simulink model "platoon"  (R2023a)
settings: Solver=VariableStepAuto  StartTime=0.0  StopTime=50  RelTol=1e-3
values from neighbouring files (symbols this model uses):
  d_default = 0.5    [prerun.m]
  t_hw = 0.1    [prerun.m]
  td_comm = 0.1    [prerun.m]
  td_comm_leader = ones(n,1)    [prerun.m]
  td_input = 0    [prerun.m]
undefined symbols (not defined in the file or in its folder): sigbuilder_block
libraries: cstblocks x21, slpidlib x2
settings Model: Creator=ritvi  LastModifiedBy=ritvi

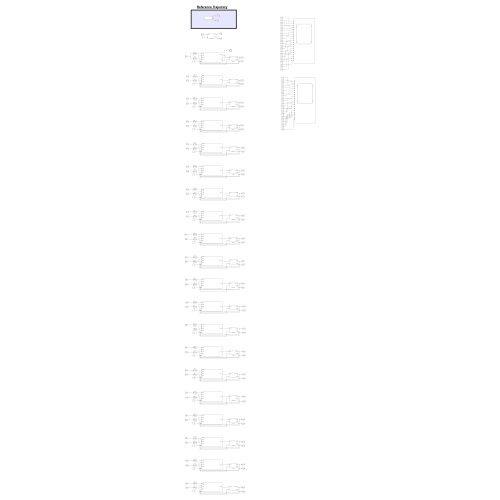
[thumbnail: Simulink's stored preview of the top-level diagram]
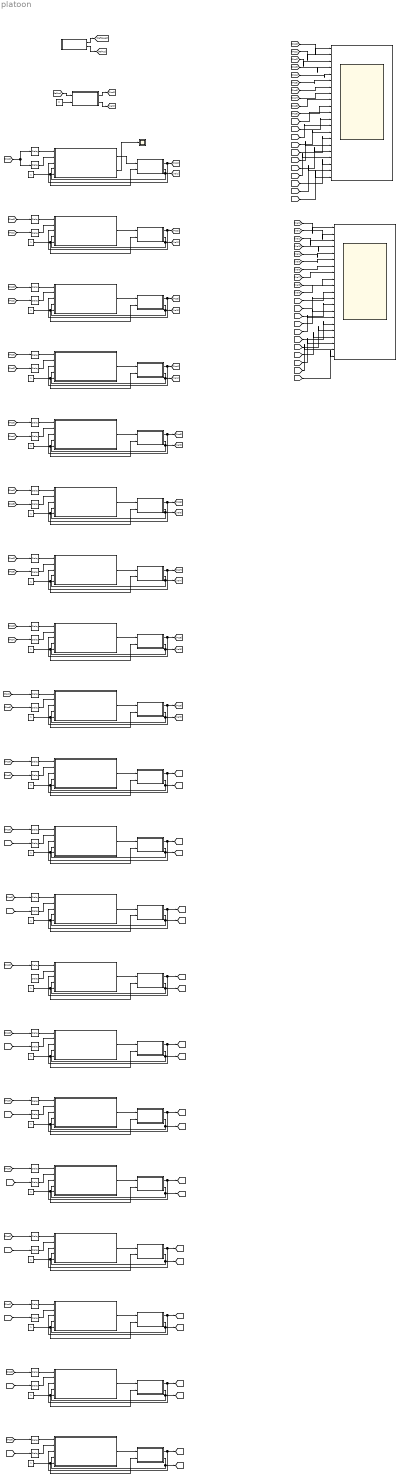
== system platoon ==
  note: Reference Trajectory
  Constant : Constant  Value=0
  Constant{1..20} (20 alike) : Constant
  Scope : Scope  NumInputPorts=21
  Scope1 : Scope  NumInputPorts=21
  Scope2 : Scope
  Subsystem : Subsystem
  Subsystem1 : Subsystem
  Subsystem10 : Subsystem
  Subsystem11 : Subsystem
  Subsystem12 : Subsystem
  Subsystem13 : Subsystem
  Subsystem14 : Subsystem
  Subsystem15 : Subsystem
  Subsystem16 : Subsystem
  Subsystem17 : Subsystem
  Subsystem18 : Subsystem
  Subsystem19 : Subsystem
  Subsystem2 : Subsystem
  Subsystem20 : Subsystem
  Subsystem3 : Subsystem
  Subsystem4 : Subsystem
  Subsystem5 : Subsystem
  Subsystem6 : Subsystem
  Subsystem7 : Subsystem
  Subsystem8 : Subsystem
  Subsystem9 : Subsystem
  Transport Delay{,2,4,6,8,10,12,14,16,18,20,22,24,26,28,30,32,34,36,38} (20 alike) : TransportDelay  DelayTime=td_comm
  Transport Delay1 : TransportDelay  DelayTime=td_comm_leader(1)
  Transport Delay11 : TransportDelay  DelayTime=td_comm_leader(6)
  Transport Delay13 : TransportDelay  DelayTime=td_comm_leader(7)
  Transport Delay15 : TransportDelay  DelayTime=td_comm_leader(8)
  Transport Delay17 : TransportDelay  DelayTime=td_comm_leader(9)
  Transport Delay19 : TransportDelay  DelayTime=td_comm_leader(10)
  Transport Delay21 : TransportDelay  DelayTime=td_comm_leader(11)
  Transport Delay23 : TransportDelay  DelayTime=td_comm_leader(12)
  Transport Delay25 : TransportDelay  DelayTime=td_comm_leader(13)
  Transport Delay27 : TransportDelay  DelayTime=td_comm_leader(14)
  Transport Delay29 : TransportDelay  DelayTime=td_comm_leader(15)
  Transport Delay3 : TransportDelay  DelayTime=td_comm_leader(2)
  Transport Delay31 : TransportDelay  DelayTime=td_comm_leader(16)
  Transport Delay33 : TransportDelay  DelayTime=td_comm_leader(17)
  Transport Delay35 : TransportDelay  DelayTime=td_comm_leader(18)
  Transport Delay37 : TransportDelay  DelayTime=td_comm_leader(19)
  Transport Delay39 : TransportDelay  DelayTime=td_comm_leader(20)
  Transport Delay5 : TransportDelay  DelayTime=td_comm_leader(3)
  Transport Delay7 : TransportDelay  DelayTime=td_comm_leader(4)
  Transport Delay9 : TransportDelay  DelayTime=td_comm_leader(5)
  Vehicle 0 : Subsystem
  Vehicle 1 : Subsystem
  Vehicle 10 : Subsystem
  Vehicle 11 : Subsystem
  Vehicle 12 : Subsystem
  Vehicle 13 : Subsystem
  Vehicle 14 : Subsystem
  Vehicle 15 : Subsystem
  Vehicle 16 : Subsystem
  Vehicle 17 : Subsystem
  Vehicle 18 : Subsystem
  Vehicle 19 : Subsystem
  Vehicle 2 : Subsystem
  Vehicle 20 : Subsystem
  Vehicle 3 : Subsystem
  Vehicle 4 : Subsystem
  Vehicle 5 : Subsystem
  Vehicle 6 : Subsystem
  Vehicle 7 : Subsystem
  Vehicle 8 : Subsystem
  Vehicle 9 : Subsystem
  wires:
  Subsystem1/1(vl) -> [RefSpeed]
  Subsystem1/2(al) -> [RefAcc]
  Subsystem/1(CmdAcc) -> Vehicle 1/1(RefAcc)
  Vehicle 1/1(position) -> [Pos1], Subsystem/3(PosEgo)
  Vehicle 1/2(speed) -> Subsystem/4(VelEgo), [Vel1]
  Constant1/1 -> Vehicle 1/2(i), Subsystem/5(i)
  Transport Delay/1 -> Subsystem/2(PosPred)
  Constant/1 -> Vehicle 0/2(i)
  [RefAcc] -> Vehicle 0/1(RefAcc)
  Vehicle 0/1(position) -> [Pos0]
  Vehicle 0/2(speed) -> [Vel0]
  Transport Delay1/1 -> Subsystem/1(PosLead)
  [Pos0] -> Transport Delay1/1, Transport Delay/1
  [Pos0] -> Transport Delay3/1
  Transport Delay2/1 -> Subsystem2/2(PosPred)
  Subsystem2/1(CmdAcc) -> Vehicle 2/1(RefAcc)
  Vehicle 2/1(position) -> [Pos2], Subsystem2/3(PosEgo)
  Vehicle 2/2(speed) -> Subsystem2/4(VelEgo), [Vel2]
  Constant2/1 -> Vehicle 2/2(i), Subsystem2/5(i)
  Transport Delay3/1 -> Subsystem2/1(PosLead)
  [Pos0] -> Transport Delay5/1
  Transport Delay4/1 -> Subsystem3/2(PosPred)
  Subsystem3/1(CmdAcc) -> Vehicle 3/1(RefAcc)
  Vehicle 3/1(position) -> [Pos3], Subsystem3/3(PosEgo)
  Vehicle 3/2(speed) -> [Vel3], Subsystem3/4(VelEgo)
  Constant3/1 -> Vehicle 3/2(i), Subsystem3/5(i)
  Transport Delay5/1 -> Subsystem3/1(PosLead)
  Vehicle 5/2(speed) -> [Vel5], Subsystem5/4(VelEgo)
  Transport Delay9/1 -> Subsystem5/1(PosLead)
  Subsystem5/1(CmdAcc) -> Vehicle 5/1(RefAcc)
  Vehicle 5/1(position) -> [Pos5], Subsystem5/3(PosEgo)
  Transport Delay8/1 -> Subsystem5/2(PosPred)
  [Pos0] -> Transport Delay9/1
  Transport Delay7/1 -> Subsystem4/1(PosLead)
  [Pos0] -> Transport Delay7/1
  Vehicle 4/2(speed) -> [Vel4], Subsystem4/4(VelEgo)
  Constant5/1 -> Vehicle 5/2(i), Subsystem5/5(i)
  Transport Delay6/1 -> Subsystem4/2(PosPred)
  Constant4/1 -> Vehicle 4/2(i), Subsystem4/5(i)
  Subsystem4/1(CmdAcc) -> Vehicle 4/1(RefAcc)
  Vehicle 4/1(position) -> Subsystem4/3(PosEgo), [Pos4]
  Vehicle 7/2(speed) -> Subsystem7/4(VelEgo), [Vel7]
  Transport Delay13/1 -> Subsystem7/1(PosLead)
  Subsystem7/1(CmdAcc) -> Vehicle 7/1(RefAcc)
  Vehicle 7/1(position) -> [Pos7], Subsystem7/3(PosEgo)
  Transport Delay12/1 -> Subsystem7/2(PosPred)
  [Pos0] -> Transport Delay13/1
  Transport Delay11/1 -> Subsystem6/1(PosLead)
  [Pos0] -> Transport Delay11/1
  Vehicle 6/2(speed) -> [Vel6], Subsystem6/4(VelEgo)
  Constant7/1 -> Vehicle 7/2(i), Subsystem7/5(i)
  Transport Delay10/1 -> Subsystem6/2(PosPred)
  Constant6/1 -> Vehicle 6/2(i), Subsystem6/5(i)
  Subsystem6/1(CmdAcc) -> Vehicle 6/1(RefAcc)
  Vehicle 6/1(position) -> [Pos6], Subsystem6/3(PosEgo)
  Vehicle 9/2(speed) -> [Vel9], Subsystem9/4(VelEgo)
  Transport Delay17/1 -> Subsystem9/1(PosLead)
  Subsystem9/1(CmdAcc) -> Vehicle 9/1(RefAcc)
  Vehicle 9/1(position) -> Subsystem9/3(PosEgo), [Pos9]
  Transport Delay16/1 -> Subsystem9/2(PosPred)
  [Pos0] -> Transport Delay17/1
  Transport Delay15/1 -> Subsystem8/1(PosLead)
  [Pos0] -> Transport Delay15/1
  Vehicle 8/2(speed) -> [Vel8], Subsystem8/4(VelEgo)
  Constant9/1 -> Vehicle 9/2(i), Subsystem9/5(i)
  Transport Delay14/1 -> Subsystem8/2(PosPred)
  Constant8/1 -> Vehicle 8/2(i), Subsystem8/5(i)
  Subsystem8/1(CmdAcc) -> Vehicle 8/1(RefAcc)
  Vehicle 8/1(position) -> [Pos8], Subsystem8/3(PosEgo)
  Vehicle 11/2(speed) -> Subsystem11/4(VelEgo), [Vel11]
  Transport Delay21/1 -> Subsystem11/1(PosLead)
  Subsystem11/1(CmdAcc) -> Vehicle 11/1(RefAcc)
  Vehicle 11/1(position) -> [Pos11], Subsystem11/3(PosEgo)
  Transport Delay20/1 -> Subsystem11/2(PosPred)
  [Pos0] -> Transport Delay21/1
  Transport Delay19/1 -> Subsystem10/1(PosLead)
  [Pos0] -> Transport Delay19/1
  Vehicle 10/2(speed) -> [Vel10], Subsystem10/4(VelEgo)
  Constant11/1 -> Vehicle 11/2(i), Subsystem11/5(i)
  Transport Delay18/1 -> Subsystem10/2(PosPred)
  Constant10/1 -> Vehicle 10/2(i), Subsystem10/5(i)
  Subsystem10/1(CmdAcc) -> Vehicle 10/1(RefAcc)
  Vehicle 10/1(position) -> [Pos10], Subsystem10/3(PosEgo)
  Vehicle 13/2(speed) -> [Vel13], Subsystem13/4(VelEgo)
  Transport Delay25/1 -> Subsystem13/1(PosLead)
  Subsystem13/1(CmdAcc) -> Vehicle 13/1(RefAcc)
  Vehicle 13/1(position) -> [Pos13], Subsystem13/3(PosEgo)
  Transport Delay24/1 -> Subsystem13/2(PosPred)
  [Pos0] -> Transport Delay25/1
  Transport Delay23/1 -> Subsystem12/1(PosLead)
  [Pos0] -> Transport Delay23/1
  Vehicle 12/2(speed) -> Subsystem12/4(VelEgo), [Vel12]
  Constant13/1 -> Vehicle 13/2(i), Subsystem13/5(i)
  Transport Delay22/1 -> Subsystem12/2(PosPred)
  Constant12/1 -> Vehicle 12/2(i), Subsystem12/5(i)
  Subsystem12/1(CmdAcc) -> Vehicle 12/1(RefAcc)
  Vehicle 12/1(position) -> [Pos12], Subsystem12/3(PosEgo)
  Vehicle 15/2(speed) -> [Vel15], Subsystem15/4(VelEgo)
  Transport Delay29/1 -> Subsystem15/1(PosLead)
  Subsystem15/1(CmdAcc) -> Vehicle 15/1(RefAcc)
  Vehicle 15/1(position) -> [Pos15], Subsystem15/3(PosEgo)
  Transport Delay28/1 -> Subsystem15/2(PosPred)
  [Pos0] -> Transport Delay29/1
  Transport Delay27/1 -> Subsystem14/1(PosLead)
  [Pos0] -> Transport Delay27/1
  Vehicle 14/2(speed) -> [Vel14], Subsystem14/4(VelEgo)
  Constant15/1 -> Vehicle 15/2(i), Subsystem15/5(i)
  Transport Delay26/1 -> Subsystem14/2(PosPred)
  Constant14/1 -> Vehicle 14/2(i), Subsystem14/5(i)
  Subsystem14/1(CmdAcc) -> Vehicle 14/1(RefAcc)
  Vehicle 14/1(position) -> Subsystem14/3(PosEgo), [Pos14]
  Vehicle 17/2(speed) -> [Vel17], Subsystem17/4(VelEgo)
  Transport Delay33/1 -> Subsystem17/1(PosLead)
  Subsystem17/1(CmdAcc) -> Vehicle 17/1(RefAcc)
  Vehicle 17/1(position) -> [Pos17], Subsystem17/3(PosEgo)
  Transport Delay32/1 -> Subsystem17/2(PosPred)
  [Pos0] -> Transport Delay33/1
  Transport Delay31/1 -> Subsystem16/1(PosLead)
  [Pos0] -> Transport Delay31/1
  Vehicle 16/2(speed) -> [Vel16], Subsystem16/4(VelEgo)
  Constant17/1 -> Vehicle 17/2(i), Subsystem17/5(i)
  Transport Delay30/1 -> Subsystem16/2(PosPred)
  Constant16/1 -> Vehicle 16/2(i), Subsystem16/5(i)
  Subsystem16/1(CmdAcc) -> Vehicle 16/1(RefAcc)
  Vehicle 16/1(position) -> [Pos16], Subsystem16/3(PosEgo)
  Vehicle 19/2(speed) -> [Vel19], Subsystem19/4(VelEgo)
  Transport Delay37/1 -> Subsystem19/1(PosLead)
  Subsystem19/1(CmdAcc) -> Vehicle 19/1(RefAcc)
  Vehicle 19/1(position) -> [Pos19], Subsystem19/3(PosEgo)
  Transport Delay36/1 -> Subsystem19/2(PosPred)
  [Pos0] -> Transport Delay37/1
  Transport Delay35/1 -> Subsystem18/1(PosLead)
  [Pos0] -> Transport Delay35/1
  Vehicle 18/2(speed) -> [Vel18], Subsystem18/4(VelEgo)
  Constant19/1 -> Vehicle 19/2(i), Subsystem19/5(i)
  Transport Delay34/1 -> Subsystem18/2(PosPred)
  Constant18/1 -> Vehicle 18/2(i), Subsystem18/5(i)
  Subsystem18/1(CmdAcc) -> Vehicle 18/1(RefAcc)
  Vehicle 18/1(position) -> [Pos18], Subsystem18/3(PosEgo)
  Vehicle 20/2(speed) -> [Vel20], Subsystem20/4(VelEgo)
  [Pos0] -> Transport Delay39/1
  Vehicle 20/1(position) -> [Pos20], Subsystem20/3(PosEgo)
  Subsystem20/1(CmdAcc) -> Vehicle 20/1(RefAcc)
  Transport Delay38/1 -> Subsystem20/2(PosPred)
  Transport Delay39/1 -> Subsystem20/1(PosLead)
  Constant20/1 -> Vehicle 20/2(i), Subsystem20/5(i)
  [Pos1] -> Transport Delay2/1
  [Pos2] -> Transport Delay4/1
  [Pos3] -> Transport Delay6/1
  [Pos4] -> Transport Delay8/1
  [Pos5] -> Transport Delay10/1
  [Pos6] -> Transport Delay12/1
  [Pos7] -> Transport Delay14/1
  [Pos8] -> Transport Delay16/1
  [Pos9] -> Transport Delay18/1
  [Pos10] -> Transport Delay20/1
  [Pos11] -> Transport Delay22/1
  [Pos13] -> Transport Delay26/1
  [Pos14] -> Transport Delay28/1
  [Pos15] -> Transport Delay30/1
  [Pos16] -> Transport Delay32/1
  [Pos17] -> Transport Delay34/1
  [Pos18] -> Transport Delay36/1
  [Pos19] -> Transport Delay38/1
  [Vel6] -> Scope1/7
  [Vel15] -> Scope1/16
  [Vel9] -> Scope1/10
  [Vel7] -> Scope1/8
  [Vel3] -> Scope1/4
  [Vel16] -> Scope1/17
  [Vel10] -> Scope1/11
  [Vel17] -> Scope1/18
  [Vel12] -> Scope1/13
  [Vel18] -> Scope1/19
  [Vel19] -> Scope1/20
  [Vel0] -> Scope1/1
  [Vel4] -> Scope1/5
  [Vel5] -> Scope1/6
  [Vel13] -> Scope1/14
  [Vel2] -> Scope1/3
  [Vel14] -> Scope1/15
  [Vel11] -> Scope1/12
  [Vel8] -> Scope1/9
  [Vel1] -> Scope1/2
  [Pos0] -> Scope/1
  [Pos1] -> Scope/2
  [Pos2] -> Scope/3
  [Pos3] -> Scope/4
  [Pos4] -> Scope/5
  [Pos5] -> Scope/6
  [Pos6] -> Scope/7
  [Pos7] -> Scope/8
  [Pos8] -> Scope/9
  [Pos9] -> Scope/10
  [Pos10] -> Scope/11
  [Pos11] -> Scope/12
  [Pos12] -> Scope/13
  [Pos13] -> Scope/14
  [Pos14] -> Scope/15
  [Pos15] -> Scope/16
  [Pos16] -> Scope/17
  [Pos17] -> Scope/18
  [Pos18] -> Scope/19
  [Pos19] -> Scope/20
  [Pos20] -> Scope/21
  [Vel20] -> Scope1/21
  Subsystem/2(dRef) -> Scope2/1

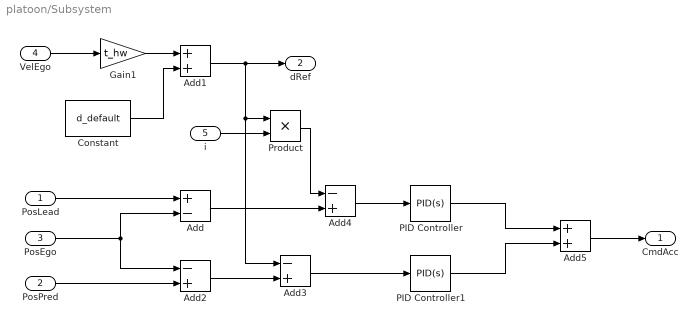
== system platoon/Subsystem ==
  PosLead : Inport
  PosPred : Inport  Port=2
  PosEgo : Inport  Port=3
  VelEgo : Inport  Port=4
  i : Inport  Port=5
  Add : Sum  Inputs=+-
  Add1 : Sum
  Add2 : Sum  Inputs=-+
  Add3 : Sum  Inputs=-+
  Add4 : Sum  Inputs=-+
  Add5 : Sum
  Constant : Constant  Value=d_default
  Gain1 : Gain  Gain=t_hw
  PID Controller : slpidlib/PID Controller  Controller=PID  Form=Parallel  TimeDomain=Continuous-time  UseExternalTs=off  SampleTime=-1  IntegratorMethod=Forward Euler  FilterMethod=Forward Euler  ControllerParametersSource=internal  P=0.576451298522446  I=0.0205713434170497  UseKiTs=off  D=3.58908348590213  N=699.068550061426  UseFilter=on  TunerSelectOption=Transfer Function Based (PID Tuner App)  InitialConditionSource=internal  InitialConditionForIntegrator=0  InitialConditionForFilter=0  DifferentiatorICPrevScaledInput=0  ExternalReset=none  TrackingMode=off  Kt=1  LimitOutput=off  SatLimitsSource=internal  UpperSaturationLimit=inf  LowerSaturationLimit=-inf  LinearizeAsGain=on  AntiWindupMode=none  Kb=1  LimitIntegrator=off  UpperIntegratorSaturationLimit=inf  LowerIntegratorSaturationLimit=-inf  POutMin=[]  POutMax=[]  IOutMin=[]  IOutMax=[]  DOutMin=[]  DOutMax=[]  NOutMin=[]  NOutMax=[]  SumOutMin=[]  SumOutMax=[]  SaturationOutMin=[]  SaturationOutMax=[]  PParamMin=[]  PParamMax=[]  IParamMin=[]  IParamMax=[]  DParamMin=[]  DParamMax=[]  NParamMin=[]  NParamMax=[]  KbParamMin=[]  KbParamMax=[]  KtParamMin=[]  KtParamMax=[]  KbOutMin=[]  KbOutMax=[]  KtOutMin=[]  KtOutMax=[]  IntegratorOutMin=[]  IntegratorOutMax=[]  FilterOutMin=[]  FilterOutMax=[]  SumI1OutMin=[]  SumI1OutMax=[]  SumI2OutMin=[]  SumI2OutMax=[]  SumI3OutMin=[]  SumI3OutMax=[]  SumI4OutMin=[]  SumI4OutMax=[]  SumDOutMin=[]  SumDOutMax=[]  DifferentiatorOutMin=[]  DifferentiatorOutMax=[]  FilterDiffOutCoefMin=[]  FilterDiffOutCoefMax=[]  ReciprocalOutMin=[]  ReciprocalOutMax=[]  SumDenOutMin=[]  SumDenOutMax=[]  SumNumOutMin=[]  SumNumOutMax=[]  DivideOutMin=[]  DivideOutMax=[]  UdiffTsProdOutMin=[]  UdiffTsProdOutMax=[]  NTsProdOutMin=[]  NTsProdOutMax=[]  UintegralTsProdOutMin=[]  UintegralTsProdOutMax=[]  UngainTsProdOutMin=[]  UngainTsProdOutMax=[]  ClampingZeroOutDataTypeStr=Inherit: Inherit via back propagation  ClampingZeroOutMin=[]  ClampingZeroOutMax=[]  FilterDenConstantOutDataTypeStr=Inherit: Inherit via back propagation  FilterDenConstantOutMin=[]  FilterDenConstantOutMax=[]  PCopyOutDataTypeStr=Inherit: Inherit via back propagation  PCopyOutMin=[]  PCopyOutMax=[]  NCopyOutDataTypeStr=Inherit: Inherit via back propagation  NCopyOutMin=[]  NCopyOutMax=[]  IntegratorContinuousStateAttributes=''  IntegratorStateMustResolveToSignalObject=off  IntegratorRTWStateStorageClass=Auto  FilterContinuousStateAttributes=''  FilterStateMustResolveToSignalObject=off  FilterRTWStateStorageClass=Auto  ParallelPVariant=InternalParameters  IdealPVariant=Disabled  IVariant=InternalParameters  DVariant=InternalParameters  IntegratorVariant=Continuous  SatVariant=Disabled  AWVariant=Passthrough  PCopyVariant=Disabled  TRVariant=Disabled  FdbkBlocksVariant=Forward  IdealPFdbkVariant=Disabled  SatFdbkVariant=Disabled  DerivativeFilterVariant=ContFilter  NVariant=InternalParameters  NCopyVariant=Disabled  FilterICVariant=InternalICsFilter  IntegratorICVariant=InternalICs  ExternalResetVariant=Disabled  TRSumVariant=Passthrough  SumFdbkVariant=Disabled  SumVariant=Sum_PID  TsampFilterVariant=InternalTs  TsampNgainVariant=Passthrough  TsampIntegralVariant=Disabled_SignalSpec  ExternalSaturationOutDataTypeStr=Inherit: Same as second input
  PID Controller1 : slpidlib/PID Controller  Controller=PID  Form=Parallel  TimeDomain=Continuous-time  UseExternalTs=off  SampleTime=-1  IntegratorMethod=Forward Euler  FilterMethod=Forward Euler  ControllerParametersSource=internal  P=2.26020185306904  I=1.23268526868394  UseKiTs=off  D=0.721287263224754  N=7.7307480132385  UseFilter=on  TunerSelectOption=Transfer Function Based (PID Tuner App)  InitialConditionSource=internal  InitialConditionForIntegrator=0  InitialConditionForFilter=0  DifferentiatorICPrevScaledInput=0  ExternalReset=none  TrackingMode=off  Kt=1  LimitOutput=off  SatLimitsSource=internal  UpperSaturationLimit=inf  LowerSaturationLimit=-inf  LinearizeAsGain=on  AntiWindupMode=none  Kb=1  LimitIntegrator=off  UpperIntegratorSaturationLimit=inf  LowerIntegratorSaturationLimit=-inf  POutMin=[]  POutMax=[]  IOutMin=[]  IOutMax=[]  DOutMin=[]  DOutMax=[]  NOutMin=[]  NOutMax=[]  SumOutMin=[]  SumOutMax=[]  SaturationOutMin=[]  SaturationOutMax=[]  PParamMin=[]  PParamMax=[]  IParamMin=[]  IParamMax=[]  DParamMin=[]  DParamMax=[]  NParamMin=[]  NParamMax=[]  KbParamMin=[]  KbParamMax=[]  KtParamMin=[]  KtParamMax=[]  KbOutMin=[]  KbOutMax=[]  KtOutMin=[]  KtOutMax=[]  IntegratorOutMin=[]  IntegratorOutMax=[]  FilterOutMin=[]  FilterOutMax=[]  SumI1OutMin=[]  SumI1OutMax=[]  SumI2OutMin=[]  SumI2OutMax=[]  SumI3OutMin=[]  SumI3OutMax=[]  SumI4OutMin=[]  SumI4OutMax=[]  SumDOutMin=[]  SumDOutMax=[]  DifferentiatorOutMin=[]  DifferentiatorOutMax=[]  FilterDiffOutCoefMin=[]  FilterDiffOutCoefMax=[]  ReciprocalOutMin=[]  ReciprocalOutMax=[]  SumDenOutMin=[]  SumDenOutMax=[]  SumNumOutMin=[]  SumNumOutMax=[]  DivideOutMin=[]  DivideOutMax=[]  UdiffTsProdOutMin=[]  UdiffTsProdOutMax=[]  NTsProdOutMin=[]  NTsProdOutMax=[]  UintegralTsProdOutMin=[]  UintegralTsProdOutMax=[]  UngainTsProdOutMin=[]  UngainTsProdOutMax=[]  ClampingZeroOutDataTypeStr=Inherit: Inherit via back propagation  ClampingZeroOutMin=[]  ClampingZeroOutMax=[]  FilterDenConstantOutDataTypeStr=Inherit: Inherit via back propagation  FilterDenConstantOutMin=[]  FilterDenConstantOutMax=[]  PCopyOutDataTypeStr=Inherit: Inherit via back propagation  PCopyOutMin=[]  PCopyOutMax=[]  NCopyOutDataTypeStr=Inherit: Inherit via back propagation  NCopyOutMin=[]  NCopyOutMax=[]  IntegratorContinuousStateAttributes=''  IntegratorStateMustResolveToSignalObject=off  IntegratorRTWStateStorageClass=Auto  FilterContinuousStateAttributes=''  FilterStateMustResolveToSignalObject=off  FilterRTWStateStorageClass=Auto  ParallelPVariant=InternalParameters  IdealPVariant=Disabled  IVariant=InternalParameters  DVariant=InternalParameters  IntegratorVariant=Continuous  SatVariant=Disabled  AWVariant=Passthrough  PCopyVariant=Disabled  TRVariant=Disabled  FdbkBlocksVariant=Forward  IdealPFdbkVariant=Disabled  SatFdbkVariant=Disabled  DerivativeFilterVariant=ContFilter  NVariant=InternalParameters  NCopyVariant=Disabled  FilterICVariant=InternalICsFilter  IntegratorICVariant=InternalICs  ExternalResetVariant=Disabled  TRSumVariant=Passthrough  SumFdbkVariant=Disabled  SumVariant=Sum_PID  TsampFilterVariant=InternalTs  TsampNgainVariant=Passthrough  TsampIntegralVariant=Disabled_SignalSpec  ExternalSaturationOutDataTypeStr=Inherit: Same as second input
  Product : Product
  CmdAcc : Outport
  dRef : Outport  Port=2
  wires:
  PosLead/1 -> Add/1
  PosEgo/1 -> Add/2, Add2/1
  VelEgo/1 -> Gain1/1
  Gain1/1 -> Add1/1
  Constant/1 -> Add1/2
  PosPred/1 -> Add2/2
  Add2/1 -> Add3/2
  Add1/1 -> dRef/1, Product/1, Add3/1
  i/1 -> Product/2
  Add/1 -> Add4/2
  Product/1 -> Add4/1
  Add4/1 -> PID Controller/1
  Add3/1 -> PID Controller1/1
  PID Controller/1 -> Add5/1
  PID Controller1/1 -> Add5/2
  Add5/1 -> CmdAcc/1

== system platoon/Subsystem1 ==
  Integrator1 : Integrator
  Scope2 : Scope
  Signal Builder New : Subsystem  Tag=STV Subsys  LoadFcn=sigbuilder_block('load');  StartFcn=sigbuilder_block('start');  StopFcn=sigbuilder_block('stop');  ClipboardFcn=sigbuilder_block('clipboard');  mask(Sigbuilder block){tuvar=[0:10]}
      mask help: Simulink:masks:SigbuilderBlock_MD
      mask init:
      | if ~strcmp(get_param(bdroot(gcbh),'SimulationStatus'),'stopped') tuvar = sigbuilder_block('maskInit'); end
      settings: CopyFcn=sigbuilder_block('copy');  DeleteFcn=sigbuilder_block('delete');  ModelCloseFcn=sigbuilder_block('modelClose');  PreSaveFcn=sigbuilder_block('preSave');  PauseFcn=sigbuilder_block('pause');  ContinueFcn=sigbuilder_block('continue');  NameChangeFcn=sigbuilder_block('namechange');  OpenFcn=sigbuilder_block('open',[485.4 187.8 550.2 361.2 ]);  CloseFcn=sigbuilder_block('close');
      mask Display: plot(0, 0, 100, 100,[2, 2, 32, 32, 2], [68, 8, 8, 68, 68],[32, 2], [38, 38], [32, 19, 2],[53, 60, 44], [32, 17, 17, 2],[16, 16, 31, 31]);txt = getActiveGroup(gcbh);text(2, 100, txt,'verticalAlignment', 'top');
  vl : Outport  VectorParamsAs1DForOutWhenUnconnected=off
  al : Outport  Port=2  VectorParamsAs1DForOutWhenUnconnected=off
  wires:
  Integrator1/1 -> Scope2/1, vl/1
  Signal Builder New/1(Signal 1) -> al/1, Integrator1/1

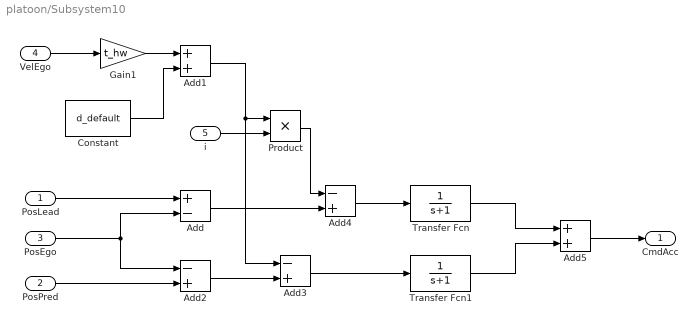
== system platoon/Subsystem10 ==
  PosLead : Inport
  PosPred : Inport  Port=2
  PosEgo : Inport  Port=3
  VelEgo : Inport  Port=4
  i : Inport  Port=5
  Add : Sum  Inputs=+-
  Add1 : Sum
  Add2 : Sum  Inputs=-+
  Add3 : Sum  Inputs=-+
  Add4 : Sum  Inputs=-+
  Add5 : Sum
  Constant : Constant  Value=d_default
  Gain1 : Gain  Gain=t_hw
  Product : Product
  Transfer Fcn : TransferFcn  Denominator=[1 1]
  Transfer Fcn1 : TransferFcn  Denominator=[1 1]
  CmdAcc : Outport
  wires:
  PosLead/1 -> Add/1
  PosEgo/1 -> Add/2, Add2/1
  VelEgo/1 -> Gain1/1
  Gain1/1 -> Add1/1
  Constant/1 -> Add1/2
  PosPred/1 -> Add2/2
  Add2/1 -> Add3/2
  Add1/1 -> Product/1, Add3/1
  i/1 -> Product/2
  Add/1 -> Add4/2
  Product/1 -> Add4/1
  Add4/1 -> Transfer Fcn/1
  Add3/1 -> Transfer Fcn1/1
  Transfer Fcn/1 -> Add5/1
  Transfer Fcn1/1 -> Add5/2
  Add5/1 -> CmdAcc/1

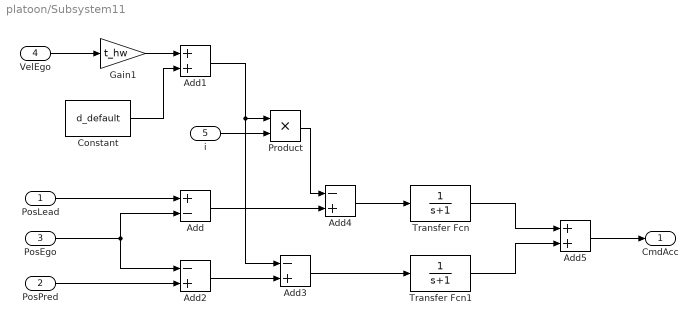
== system platoon/Subsystem11 ==
  PosLead : Inport
  PosPred : Inport  Port=2
  PosEgo : Inport  Port=3
  VelEgo : Inport  Port=4
  i : Inport  Port=5
  Add : Sum  Inputs=+-
  Add1 : Sum
  Add2 : Sum  Inputs=-+
  Add3 : Sum  Inputs=-+
  Add4 : Sum  Inputs=-+
  Add5 : Sum
  Constant : Constant  Value=d_default
  Gain1 : Gain  Gain=t_hw
  Product : Product
  Transfer Fcn : TransferFcn  Denominator=[1 1]
  Transfer Fcn1 : TransferFcn  Denominator=[1 1]
  CmdAcc : Outport
  wires:
  PosLead/1 -> Add/1
  PosEgo/1 -> Add/2, Add2/1
  VelEgo/1 -> Gain1/1
  Gain1/1 -> Add1/1
  Constant/1 -> Add1/2
  PosPred/1 -> Add2/2
  Add2/1 -> Add3/2
  Add1/1 -> Product/1, Add3/1
  i/1 -> Product/2
  Add/1 -> Add4/2
  Product/1 -> Add4/1
  Add4/1 -> Transfer Fcn/1
  Add3/1 -> Transfer Fcn1/1
  Transfer Fcn/1 -> Add5/1
  Transfer Fcn1/1 -> Add5/2
  Add5/1 -> CmdAcc/1

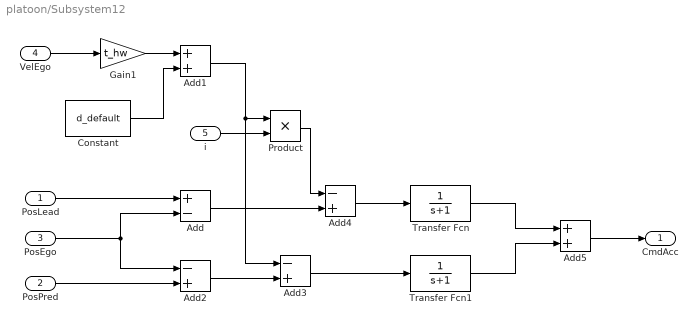
== system platoon/Subsystem12 ==
  PosLead : Inport
  PosPred : Inport  Port=2
  PosEgo : Inport  Port=3
  VelEgo : Inport  Port=4
  i : Inport  Port=5
  Add : Sum  Inputs=+-
  Add1 : Sum
  Add2 : Sum  Inputs=-+
  Add3 : Sum  Inputs=-+
  Add4 : Sum  Inputs=-+
  Add5 : Sum
  Constant : Constant  Value=d_default
  Gain1 : Gain  Gain=t_hw
  Product : Product
  Transfer Fcn : TransferFcn  Denominator=[1 1]
  Transfer Fcn1 : TransferFcn  Denominator=[1 1]
  CmdAcc : Outport
  wires:
  PosLead/1 -> Add/1
  PosEgo/1 -> Add/2, Add2/1
  VelEgo/1 -> Gain1/1
  Gain1/1 -> Add1/1
  Constant/1 -> Add1/2
  PosPred/1 -> Add2/2
  Add2/1 -> Add3/2
  Add1/1 -> Product/1, Add3/1
  i/1 -> Product/2
  Add/1 -> Add4/2
  Product/1 -> Add4/1
  Add4/1 -> Transfer Fcn/1
  Add3/1 -> Transfer Fcn1/1
  Transfer Fcn/1 -> Add5/1
  Transfer Fcn1/1 -> Add5/2
  Add5/1 -> CmdAcc/1

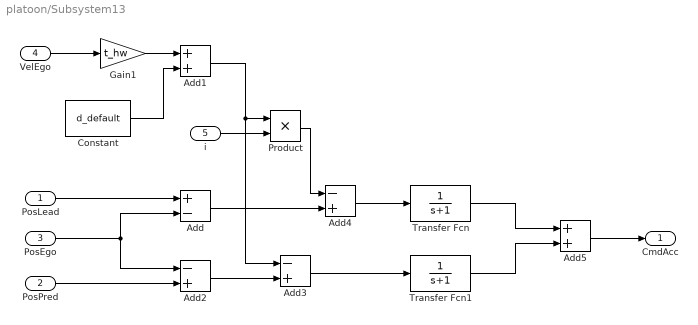
== system platoon/Subsystem13 ==
  PosLead : Inport
  PosPred : Inport  Port=2
  PosEgo : Inport  Port=3
  VelEgo : Inport  Port=4
  i : Inport  Port=5
  Add : Sum  Inputs=+-
  Add1 : Sum
  Add2 : Sum  Inputs=-+
  Add3 : Sum  Inputs=-+
  Add4 : Sum  Inputs=-+
  Add5 : Sum
  Constant : Constant  Value=d_default
  Gain1 : Gain  Gain=t_hw
  Product : Product
  Transfer Fcn : TransferFcn  Denominator=[1 1]
  Transfer Fcn1 : TransferFcn  Denominator=[1 1]
  CmdAcc : Outport
  wires:
  PosLead/1 -> Add/1
  PosEgo/1 -> Add/2, Add2/1
  VelEgo/1 -> Gain1/1
  Gain1/1 -> Add1/1
  Constant/1 -> Add1/2
  PosPred/1 -> Add2/2
  Add2/1 -> Add3/2
  Add1/1 -> Product/1, Add3/1
  i/1 -> Product/2
  Add/1 -> Add4/2
  Product/1 -> Add4/1
  Add4/1 -> Transfer Fcn/1
  Add3/1 -> Transfer Fcn1/1
  Transfer Fcn/1 -> Add5/1
  Transfer Fcn1/1 -> Add5/2
  Add5/1 -> CmdAcc/1

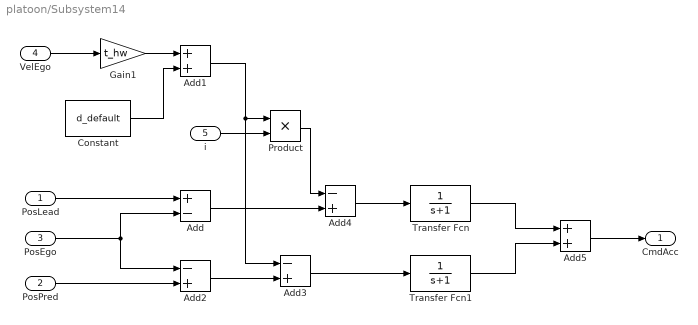
== system platoon/Subsystem14 ==
  PosLead : Inport
  PosPred : Inport  Port=2
  PosEgo : Inport  Port=3
  VelEgo : Inport  Port=4
  i : Inport  Port=5
  Add : Sum  Inputs=+-
  Add1 : Sum
  Add2 : Sum  Inputs=-+
  Add3 : Sum  Inputs=-+
  Add4 : Sum  Inputs=-+
  Add5 : Sum
  Constant : Constant  Value=d_default
  Gain1 : Gain  Gain=t_hw
  Product : Product
  Transfer Fcn : TransferFcn  Denominator=[1 1]
  Transfer Fcn1 : TransferFcn  Denominator=[1 1]
  CmdAcc : Outport
  wires:
  PosLead/1 -> Add/1
  PosEgo/1 -> Add/2, Add2/1
  VelEgo/1 -> Gain1/1
  Gain1/1 -> Add1/1
  Constant/1 -> Add1/2
  PosPred/1 -> Add2/2
  Add2/1 -> Add3/2
  Add1/1 -> Product/1, Add3/1
  i/1 -> Product/2
  Add/1 -> Add4/2
  Product/1 -> Add4/1
  Add4/1 -> Transfer Fcn/1
  Add3/1 -> Transfer Fcn1/1
  Transfer Fcn/1 -> Add5/1
  Transfer Fcn1/1 -> Add5/2
  Add5/1 -> CmdAcc/1

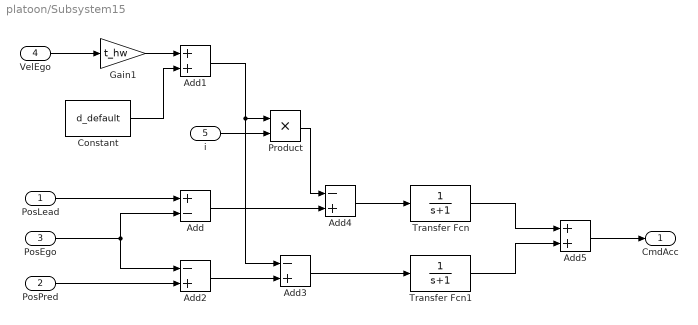
== system platoon/Subsystem15 ==
  PosLead : Inport
  PosPred : Inport  Port=2
  PosEgo : Inport  Port=3
  VelEgo : Inport  Port=4
  i : Inport  Port=5
  Add : Sum  Inputs=+-
  Add1 : Sum
  Add2 : Sum  Inputs=-+
  Add3 : Sum  Inputs=-+
  Add4 : Sum  Inputs=-+
  Add5 : Sum
  Constant : Constant  Value=d_default
  Gain1 : Gain  Gain=t_hw
  Product : Product
  Transfer Fcn : TransferFcn  Denominator=[1 1]
  Transfer Fcn1 : TransferFcn  Denominator=[1 1]
  CmdAcc : Outport
  wires:
  PosLead/1 -> Add/1
  PosEgo/1 -> Add/2, Add2/1
  VelEgo/1 -> Gain1/1
  Gain1/1 -> Add1/1
  Constant/1 -> Add1/2
  PosPred/1 -> Add2/2
  Add2/1 -> Add3/2
  Add1/1 -> Product/1, Add3/1
  i/1 -> Product/2
  Add/1 -> Add4/2
  Product/1 -> Add4/1
  Add4/1 -> Transfer Fcn/1
  Add3/1 -> Transfer Fcn1/1
  Transfer Fcn/1 -> Add5/1
  Transfer Fcn1/1 -> Add5/2
  Add5/1 -> CmdAcc/1

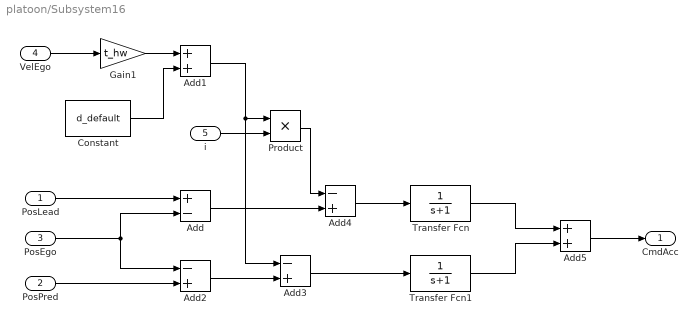
== system platoon/Subsystem16 ==
  PosLead : Inport
  PosPred : Inport  Port=2
  PosEgo : Inport  Port=3
  VelEgo : Inport  Port=4
  i : Inport  Port=5
  Add : Sum  Inputs=+-
  Add1 : Sum
  Add2 : Sum  Inputs=-+
  Add3 : Sum  Inputs=-+
  Add4 : Sum  Inputs=-+
  Add5 : Sum
  Constant : Constant  Value=d_default
  Gain1 : Gain  Gain=t_hw
  Product : Product
  Transfer Fcn : TransferFcn  Denominator=[1 1]
  Transfer Fcn1 : TransferFcn  Denominator=[1 1]
  CmdAcc : Outport
  wires:
  PosLead/1 -> Add/1
  PosEgo/1 -> Add/2, Add2/1
  VelEgo/1 -> Gain1/1
  Gain1/1 -> Add1/1
  Constant/1 -> Add1/2
  PosPred/1 -> Add2/2
  Add2/1 -> Add3/2
  Add1/1 -> Product/1, Add3/1
  i/1 -> Product/2
  Add/1 -> Add4/2
  Product/1 -> Add4/1
  Add4/1 -> Transfer Fcn/1
  Add3/1 -> Transfer Fcn1/1
  Transfer Fcn/1 -> Add5/1
  Transfer Fcn1/1 -> Add5/2
  Add5/1 -> CmdAcc/1

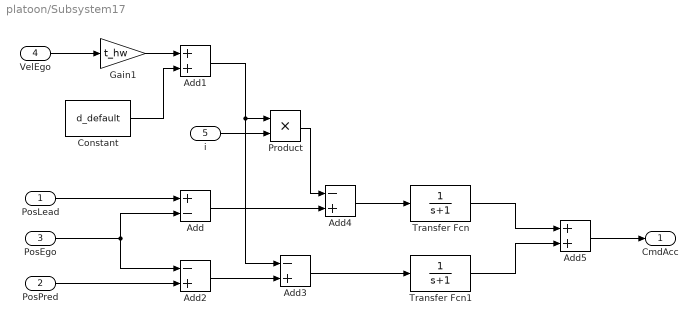
== system platoon/Subsystem17 ==
  PosLead : Inport
  PosPred : Inport  Port=2
  PosEgo : Inport  Port=3
  VelEgo : Inport  Port=4
  i : Inport  Port=5
  Add : Sum  Inputs=+-
  Add1 : Sum
  Add2 : Sum  Inputs=-+
  Add3 : Sum  Inputs=-+
  Add4 : Sum  Inputs=-+
  Add5 : Sum
  Constant : Constant  Value=d_default
  Gain1 : Gain  Gain=t_hw
  Product : Product
  Transfer Fcn : TransferFcn  Denominator=[1 1]
  Transfer Fcn1 : TransferFcn  Denominator=[1 1]
  CmdAcc : Outport
  wires:
  PosLead/1 -> Add/1
  PosEgo/1 -> Add/2, Add2/1
  VelEgo/1 -> Gain1/1
  Gain1/1 -> Add1/1
  Constant/1 -> Add1/2
  PosPred/1 -> Add2/2
  Add2/1 -> Add3/2
  Add1/1 -> Product/1, Add3/1
  i/1 -> Product/2
  Add/1 -> Add4/2
  Product/1 -> Add4/1
  Add4/1 -> Transfer Fcn/1
  Add3/1 -> Transfer Fcn1/1
  Transfer Fcn/1 -> Add5/1
  Transfer Fcn1/1 -> Add5/2
  Add5/1 -> CmdAcc/1

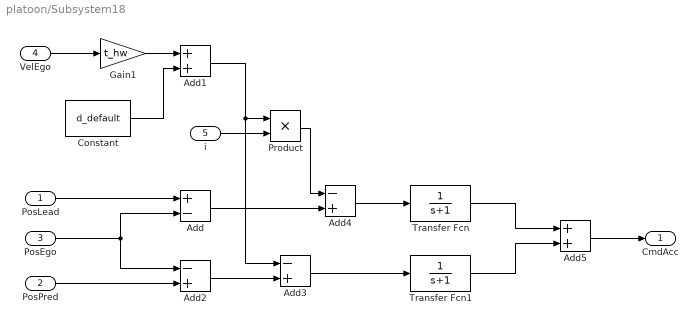
== system platoon/Subsystem18 ==
  PosLead : Inport
  PosPred : Inport  Port=2
  PosEgo : Inport  Port=3
  VelEgo : Inport  Port=4
  i : Inport  Port=5
  Add : Sum  Inputs=+-
  Add1 : Sum
  Add2 : Sum  Inputs=-+
  Add3 : Sum  Inputs=-+
  Add4 : Sum  Inputs=-+
  Add5 : Sum
  Constant : Constant  Value=d_default
  Gain1 : Gain  Gain=t_hw
  Product : Product
  Transfer Fcn : TransferFcn  Denominator=[1 1]
  Transfer Fcn1 : TransferFcn  Denominator=[1 1]
  CmdAcc : Outport
  wires:
  PosLead/1 -> Add/1
  PosEgo/1 -> Add/2, Add2/1
  VelEgo/1 -> Gain1/1
  Gain1/1 -> Add1/1
  Constant/1 -> Add1/2
  PosPred/1 -> Add2/2
  Add2/1 -> Add3/2
  Add1/1 -> Product/1, Add3/1
  i/1 -> Product/2
  Add/1 -> Add4/2
  Product/1 -> Add4/1
  Add4/1 -> Transfer Fcn/1
  Add3/1 -> Transfer Fcn1/1
  Transfer Fcn/1 -> Add5/1
  Transfer Fcn1/1 -> Add5/2
  Add5/1 -> CmdAcc/1

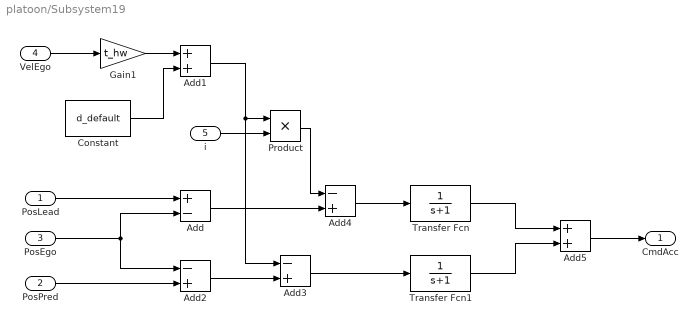
== system platoon/Subsystem19 ==
  PosLead : Inport
  PosPred : Inport  Port=2
  PosEgo : Inport  Port=3
  VelEgo : Inport  Port=4
  i : Inport  Port=5
  Add : Sum  Inputs=+-
  Add1 : Sum
  Add2 : Sum  Inputs=-+
  Add3 : Sum  Inputs=-+
  Add4 : Sum  Inputs=-+
  Add5 : Sum
  Constant : Constant  Value=d_default
  Gain1 : Gain  Gain=t_hw
  Product : Product
  Transfer Fcn : TransferFcn  Denominator=[1 1]
  Transfer Fcn1 : TransferFcn  Denominator=[1 1]
  CmdAcc : Outport
  wires:
  PosLead/1 -> Add/1
  PosEgo/1 -> Add/2, Add2/1
  VelEgo/1 -> Gain1/1
  Gain1/1 -> Add1/1
  Constant/1 -> Add1/2
  PosPred/1 -> Add2/2
  Add2/1 -> Add3/2
  Add1/1 -> Product/1, Add3/1
  i/1 -> Product/2
  Add/1 -> Add4/2
  Product/1 -> Add4/1
  Add4/1 -> Transfer Fcn/1
  Add3/1 -> Transfer Fcn1/1
  Transfer Fcn/1 -> Add5/1
  Transfer Fcn1/1 -> Add5/2
  Add5/1 -> CmdAcc/1

== system platoon/Subsystem2 ==
  PosLead : Inport
  PosPred : Inport  Port=2
  PosEgo : Inport  Port=3
  VelEgo : Inport  Port=4
  i : Inport  Port=5
  Add : Sum  Inputs=+-
  Add1 : Sum
  Add2 : Sum  Inputs=-+
  Add3 : Sum  Inputs=-+
  Add4 : Sum  Inputs=-+
  Add5 : Sum
  Constant : Constant  Value=d_default
  Gain1 : Gain  Gain=t_hw
  Product : Product
  Transfer Fcn : TransferFcn  Denominator=[1 1]
  Transfer Fcn1 : TransferFcn  Denominator=[1 1]
  CmdAcc : Outport
  wires:
  PosLead/1 -> Add/1
  PosEgo/1 -> Add/2, Add2/1
  VelEgo/1 -> Gain1/1
  Gain1/1 -> Add1/1
  Constant/1 -> Add1/2
  PosPred/1 -> Add2/2
  Add2/1 -> Add3/2
  Add1/1 -> Product/1, Add3/1
  i/1 -> Product/2
  Add/1 -> Add4/2
  Product/1 -> Add4/1
  Add4/1 -> Transfer Fcn/1
  Add3/1 -> Transfer Fcn1/1
  Transfer Fcn/1 -> Add5/1
  Transfer Fcn1/1 -> Add5/2
  Add5/1 -> CmdAcc/1

== system platoon/Subsystem20 ==
  PosLead : Inport
  PosPred : Inport  Port=2
  PosEgo : Inport  Port=3
  VelEgo : Inport  Port=4
  i : Inport  Port=5
  Add : Sum  Inputs=+-
  Add1 : Sum
  Add2 : Sum  Inputs=-+
  Add3 : Sum  Inputs=-+
  Add4 : Sum  Inputs=-+
  Add5 : Sum
  Constant : Constant  Value=d_default
  Gain1 : Gain  Gain=t_hw
  Product : Product
  Transfer Fcn : TransferFcn  Denominator=[1 1]
  Transfer Fcn1 : TransferFcn  Denominator=[1 1]
  CmdAcc : Outport
  wires:
  PosLead/1 -> Add/1
  PosEgo/1 -> Add/2, Add2/1
  VelEgo/1 -> Gain1/1
  Gain1/1 -> Add1/1
  Constant/1 -> Add1/2
  PosPred/1 -> Add2/2
  Add2/1 -> Add3/2
  Add1/1 -> Product/1, Add3/1
  i/1 -> Product/2
  Add/1 -> Add4/2
  Product/1 -> Add4/1
  Add4/1 -> Transfer Fcn/1
  Add3/1 -> Transfer Fcn1/1
  Transfer Fcn/1 -> Add5/1
  Transfer Fcn1/1 -> Add5/2
  Add5/1 -> CmdAcc/1

== system platoon/Subsystem3 ==
  PosLead : Inport
  PosPred : Inport  Port=2
  PosEgo : Inport  Port=3
  VelEgo : Inport  Port=4
  i : Inport  Port=5
  Add : Sum  Inputs=+-
  Add1 : Sum
  Add2 : Sum  Inputs=-+
  Add3 : Sum  Inputs=-+
  Add4 : Sum  Inputs=-+
  Add5 : Sum
  Constant : Constant  Value=d_default
  Gain1 : Gain  Gain=t_hw
  Product : Product
  Transfer Fcn : TransferFcn  Denominator=[1 1]
  Transfer Fcn1 : TransferFcn  Denominator=[1 1]
  CmdAcc : Outport
  wires:
  PosLead/1 -> Add/1
  PosEgo/1 -> Add/2, Add2/1
  VelEgo/1 -> Gain1/1
  Gain1/1 -> Add1/1
  Constant/1 -> Add1/2
  PosPred/1 -> Add2/2
  Add2/1 -> Add3/2
  Add1/1 -> Product/1, Add3/1
  i/1 -> Product/2
  Add/1 -> Add4/2
  Product/1 -> Add4/1
  Add4/1 -> Transfer Fcn/1
  Add3/1 -> Transfer Fcn1/1
  Transfer Fcn/1 -> Add5/1
  Transfer Fcn1/1 -> Add5/2
  Add5/1 -> CmdAcc/1

== system platoon/Subsystem4 ==
  PosLead : Inport
  PosPred : Inport  Port=2
  PosEgo : Inport  Port=3
  VelEgo : Inport  Port=4
  i : Inport  Port=5
  Add : Sum  Inputs=+-
  Add1 : Sum
  Add2 : Sum  Inputs=-+
  Add3 : Sum  Inputs=-+
  Add4 : Sum  Inputs=-+
  Add5 : Sum
  Constant : Constant  Value=d_default
  Gain1 : Gain  Gain=t_hw
  Product : Product
  Transfer Fcn : TransferFcn  Denominator=[1 1]
  Transfer Fcn1 : TransferFcn  Denominator=[1 1]
  CmdAcc : Outport
  wires:
  PosLead/1 -> Add/1
  PosEgo/1 -> Add/2, Add2/1
  VelEgo/1 -> Gain1/1
  Gain1/1 -> Add1/1
  Constant/1 -> Add1/2
  PosPred/1 -> Add2/2
  Add2/1 -> Add3/2
  Add1/1 -> Product/1, Add3/1
  i/1 -> Product/2
  Add/1 -> Add4/2
  Product/1 -> Add4/1
  Add4/1 -> Transfer Fcn/1
  Add3/1 -> Transfer Fcn1/1
  Transfer Fcn/1 -> Add5/1
  Transfer Fcn1/1 -> Add5/2
  Add5/1 -> CmdAcc/1

== system platoon/Subsystem5 ==
  PosLead : Inport
  PosPred : Inport  Port=2
  PosEgo : Inport  Port=3
  VelEgo : Inport  Port=4
  i : Inport  Port=5
  Add : Sum  Inputs=+-
  Add1 : Sum
  Add2 : Sum  Inputs=-+
  Add3 : Sum  Inputs=-+
  Add4 : Sum  Inputs=-+
  Add5 : Sum
  Constant : Constant  Value=d_default
  Gain1 : Gain  Gain=t_hw
  Product : Product
  Transfer Fcn : TransferFcn  Denominator=[1 1]
  Transfer Fcn1 : TransferFcn  Denominator=[1 1]
  CmdAcc : Outport
  wires:
  PosLead/1 -> Add/1
  PosEgo/1 -> Add/2, Add2/1
  VelEgo/1 -> Gain1/1
  Gain1/1 -> Add1/1
  Constant/1 -> Add1/2
  PosPred/1 -> Add2/2
  Add2/1 -> Add3/2
  Add1/1 -> Product/1, Add3/1
  i/1 -> Product/2
  Add/1 -> Add4/2
  Product/1 -> Add4/1
  Add4/1 -> Transfer Fcn/1
  Add3/1 -> Transfer Fcn1/1
  Transfer Fcn/1 -> Add5/1
  Transfer Fcn1/1 -> Add5/2
  Add5/1 -> CmdAcc/1

== system platoon/Subsystem6 ==
  PosLead : Inport
  PosPred : Inport  Port=2
  PosEgo : Inport  Port=3
  VelEgo : Inport  Port=4
  i : Inport  Port=5
  Add : Sum  Inputs=+-
  Add1 : Sum
  Add2 : Sum  Inputs=-+
  Add3 : Sum  Inputs=-+
  Add4 : Sum  Inputs=-+
  Add5 : Sum
  Constant : Constant  Value=d_default
  Gain1 : Gain  Gain=t_hw
  Product : Product
  Transfer Fcn : TransferFcn  Denominator=[1 1]
  Transfer Fcn1 : TransferFcn  Denominator=[1 1]
  CmdAcc : Outport
  wires:
  PosLead/1 -> Add/1
  PosEgo/1 -> Add/2, Add2/1
  VelEgo/1 -> Gain1/1
  Gain1/1 -> Add1/1
  Constant/1 -> Add1/2
  PosPred/1 -> Add2/2
  Add2/1 -> Add3/2
  Add1/1 -> Product/1, Add3/1
  i/1 -> Product/2
  Add/1 -> Add4/2
  Product/1 -> Add4/1
  Add4/1 -> Transfer Fcn/1
  Add3/1 -> Transfer Fcn1/1
  Transfer Fcn/1 -> Add5/1
  Transfer Fcn1/1 -> Add5/2
  Add5/1 -> CmdAcc/1

== system platoon/Subsystem7 ==
  PosLead : Inport
  PosPred : Inport  Port=2
  PosEgo : Inport  Port=3
  VelEgo : Inport  Port=4
  i : Inport  Port=5
  Add : Sum  Inputs=+-
  Add1 : Sum
  Add2 : Sum  Inputs=-+
  Add3 : Sum  Inputs=-+
  Add4 : Sum  Inputs=-+
  Add5 : Sum
  Constant : Constant  Value=d_default
  Gain1 : Gain  Gain=t_hw
  Product : Product
  Transfer Fcn : TransferFcn  Denominator=[1 1]
  Transfer Fcn1 : TransferFcn  Denominator=[1 1]
  CmdAcc : Outport
  wires:
  PosLead/1 -> Add/1
  PosEgo/1 -> Add/2, Add2/1
  VelEgo/1 -> Gain1/1
  Gain1/1 -> Add1/1
  Constant/1 -> Add1/2
  PosPred/1 -> Add2/2
  Add2/1 -> Add3/2
  Add1/1 -> Product/1, Add3/1
  i/1 -> Product/2
  Add/1 -> Add4/2
  Product/1 -> Add4/1
  Add4/1 -> Transfer Fcn/1
  Add3/1 -> Transfer Fcn1/1
  Transfer Fcn/1 -> Add5/1
  Transfer Fcn1/1 -> Add5/2
  Add5/1 -> CmdAcc/1

== system platoon/Subsystem8 ==
  PosLead : Inport
  PosPred : Inport  Port=2
  PosEgo : Inport  Port=3
  VelEgo : Inport  Port=4
  i : Inport  Port=5
  Add : Sum  Inputs=+-
  Add1 : Sum
  Add2 : Sum  Inputs=-+
  Add3 : Sum  Inputs=-+
  Add4 : Sum  Inputs=-+
  Add5 : Sum
  Constant : Constant  Value=d_default
  Gain1 : Gain  Gain=t_hw
  Product : Product
  Transfer Fcn : TransferFcn  Denominator=[1 1]
  Transfer Fcn1 : TransferFcn  Denominator=[1 1]
  CmdAcc : Outport
  wires:
  PosLead/1 -> Add/1
  PosEgo/1 -> Add/2, Add2/1
  VelEgo/1 -> Gain1/1
  Gain1/1 -> Add1/1
  Constant/1 -> Add1/2
  PosPred/1 -> Add2/2
  Add2/1 -> Add3/2
  Add1/1 -> Product/1, Add3/1
  i/1 -> Product/2
  Add/1 -> Add4/2
  Product/1 -> Add4/1
  Add4/1 -> Transfer Fcn/1
  Add3/1 -> Transfer Fcn1/1
  Transfer Fcn/1 -> Add5/1
  Transfer Fcn1/1 -> Add5/2
  Add5/1 -> CmdAcc/1

== system platoon/Subsystem9 ==
  PosLead : Inport
  PosPred : Inport  Port=2
  PosEgo : Inport  Port=3
  VelEgo : Inport  Port=4
  i : Inport  Port=5
  Add : Sum  Inputs=+-
  Add1 : Sum
  Add2 : Sum  Inputs=-+
  Add3 : Sum  Inputs=-+
  Add4 : Sum  Inputs=-+
  Add5 : Sum
  Constant : Constant  Value=d_default
  Gain1 : Gain  Gain=t_hw
  Product : Product
  Transfer Fcn : TransferFcn  Denominator=[1 1]
  Transfer Fcn1 : TransferFcn  Denominator=[1 1]
  CmdAcc : Outport
  wires:
  PosLead/1 -> Add/1
  PosEgo/1 -> Add/2, Add2/1
  VelEgo/1 -> Gain1/1
  Gain1/1 -> Add1/1
  Constant/1 -> Add1/2
  PosPred/1 -> Add2/2
  Add2/1 -> Add3/2
  Add1/1 -> Product/1, Add3/1
  i/1 -> Product/2
  Add/1 -> Add4/2
  Product/1 -> Add4/1
  Add4/1 -> Transfer Fcn/1
  Add3/1 -> Transfer Fcn1/1
  Transfer Fcn/1 -> Add5/1
  Transfer Fcn1/1 -> Add5/2
  Add5/1 -> CmdAcc/1

== system platoon/Vehicle 0 ==
  RefAcc : Inport
  i : Inport  Port=2
  Gain : Gain  Gain=-1*d_default
  Integrator : Integrator  InitialConditionSource=external
  Scope : Scope  NumInputPorts=2
  TF model : cstblocks/LTI System  sys=G4  IC=[]
  Transfer Fcn : TransferFcn  Denominator=[td_input 1 0]
  position : Outport
  speed : Outport  Port=2
  wires:
  TF model/1 -> Integrator/1, Scope/2, speed/1
  Integrator/1 -> position/1
  i/1 -> Gain/1
  Gain/1 -> Integrator/2
  RefAcc/1 -> Transfer Fcn/1
  Transfer Fcn/1 -> Scope/1, TF model/1

== system platoon/Vehicle 1 ==
  RefAcc : Inport
  i : Inport  Port=2
  Gain : Gain  Gain=-1*d_default
  Integrator : Integrator  InitialConditionSource=external
  TF model : cstblocks/LTI System  sys=G4  IC=[]
  Transfer Fcn : TransferFcn  Denominator=[td_input 1 0]
  position : Outport
  speed : Outport  Port=2
  wires:
  TF model/1 -> Integrator/1, speed/1
  Integrator/1 -> position/1
  i/1 -> Gain/1
  Gain/1 -> Integrator/2
  RefAcc/1 -> Transfer Fcn/1
  Transfer Fcn/1 -> TF model/1

== system platoon/Vehicle 10 ==
  RefAcc : Inport
  i : Inport  Port=2
  Gain : Gain  Gain=-1*d_default
  Integrator : Integrator  InitialConditionSource=external
  TF model : cstblocks/LTI System  sys=G4  IC=[]
  Transfer Fcn : TransferFcn  Denominator=[td_input 1 0]
  position : Outport
  speed : Outport  Port=2
  wires:
  TF model/1 -> Integrator/1, speed/1
  Integrator/1 -> position/1
  i/1 -> Gain/1
  Gain/1 -> Integrator/2
  RefAcc/1 -> Transfer Fcn/1
  Transfer Fcn/1 -> TF model/1

== system platoon/Vehicle 11 ==
  RefAcc : Inport
  i : Inport  Port=2
  Gain : Gain  Gain=-1*d_default
  Integrator : Integrator  InitialConditionSource=external
  TF model : cstblocks/LTI System  sys=G4  IC=[]
  Transfer Fcn : TransferFcn  Denominator=[td_input 1 0]
  position : Outport
  speed : Outport  Port=2
  wires:
  TF model/1 -> Integrator/1, speed/1
  Integrator/1 -> position/1
  i/1 -> Gain/1
  Gain/1 -> Integrator/2
  RefAcc/1 -> Transfer Fcn/1
  Transfer Fcn/1 -> TF model/1

== system platoon/Vehicle 12 ==
  RefAcc : Inport
  i : Inport  Port=2
  Gain : Gain  Gain=-1*d_default
  Integrator : Integrator  InitialConditionSource=external
  TF model : cstblocks/LTI System  sys=G4  IC=[]
  Transfer Fcn : TransferFcn  Denominator=[td_input 1 0]
  position : Outport
  speed : Outport  Port=2
  wires:
  TF model/1 -> Integrator/1, speed/1
  Integrator/1 -> position/1
  i/1 -> Gain/1
  Gain/1 -> Integrator/2
  RefAcc/1 -> Transfer Fcn/1
  Transfer Fcn/1 -> TF model/1

== system platoon/Vehicle 13 ==
  RefAcc : Inport
  i : Inport  Port=2
  Gain : Gain  Gain=-1*d_default
  Integrator : Integrator  InitialConditionSource=external
  TF model : cstblocks/LTI System  sys=G4  IC=[]
  Transfer Fcn : TransferFcn  Denominator=[td_input 1 0]
  position : Outport
  speed : Outport  Port=2
  wires:
  TF model/1 -> Integrator/1, speed/1
  Integrator/1 -> position/1
  i/1 -> Gain/1
  Gain/1 -> Integrator/2
  RefAcc/1 -> Transfer Fcn/1
  Transfer Fcn/1 -> TF model/1

== system platoon/Vehicle 14 ==
  RefAcc : Inport
  i : Inport  Port=2
  Gain : Gain  Gain=-1*d_default
  Integrator : Integrator  InitialConditionSource=external
  TF model : cstblocks/LTI System  sys=G4  IC=[]
  Transfer Fcn : TransferFcn  Denominator=[td_input 1 0]
  position : Outport
  speed : Outport  Port=2
  wires:
  TF model/1 -> Integrator/1, speed/1
  Integrator/1 -> position/1
  i/1 -> Gain/1
  Gain/1 -> Integrator/2
  RefAcc/1 -> Transfer Fcn/1
  Transfer Fcn/1 -> TF model/1

== system platoon/Vehicle 15 ==
  RefAcc : Inport
  i : Inport  Port=2
  Gain : Gain  Gain=-1*d_default
  Integrator : Integrator  InitialConditionSource=external
  TF model : cstblocks/LTI System  sys=G4  IC=[]
  Transfer Fcn : TransferFcn  Denominator=[td_input 1 0]
  position : Outport
  speed : Outport  Port=2
  wires:
  TF model/1 -> Integrator/1, speed/1
  Integrator/1 -> position/1
  i/1 -> Gain/1
  Gain/1 -> Integrator/2
  RefAcc/1 -> Transfer Fcn/1
  Transfer Fcn/1 -> TF model/1

== system platoon/Vehicle 16 ==
  RefAcc : Inport
  i : Inport  Port=2
  Gain : Gain  Gain=-1*d_default
  Integrator : Integrator  InitialConditionSource=external
  TF model : cstblocks/LTI System  sys=G4  IC=[]
  Transfer Fcn : TransferFcn  Denominator=[td_input 1 0]
  position : Outport
  speed : Outport  Port=2
  wires:
  TF model/1 -> Integrator/1, speed/1
  Integrator/1 -> position/1
  i/1 -> Gain/1
  Gain/1 -> Integrator/2
  RefAcc/1 -> Transfer Fcn/1
  Transfer Fcn/1 -> TF model/1

== system platoon/Vehicle 17 ==
  RefAcc : Inport
  i : Inport  Port=2
  Gain : Gain  Gain=-1*d_default
  Integrator : Integrator  InitialConditionSource=external
  TF model : cstblocks/LTI System  sys=G4  IC=[]
  Transfer Fcn : TransferFcn  Denominator=[td_input 1 0]
  position : Outport
  speed : Outport  Port=2
  wires:
  TF model/1 -> Integrator/1, speed/1
  Integrator/1 -> position/1
  i/1 -> Gain/1
  Gain/1 -> Integrator/2
  RefAcc/1 -> Transfer Fcn/1
  Transfer Fcn/1 -> TF model/1

== system platoon/Vehicle 18 ==
  RefAcc : Inport
  i : Inport  Port=2
  Gain : Gain  Gain=-1*d_default
  Integrator : Integrator  InitialConditionSource=external
  TF model : cstblocks/LTI System  sys=G4  IC=[]
  Transfer Fcn : TransferFcn  Denominator=[td_input 1 0]
  position : Outport
  speed : Outport  Port=2
  wires:
  TF model/1 -> Integrator/1, speed/1
  Integrator/1 -> position/1
  i/1 -> Gain/1
  Gain/1 -> Integrator/2
  RefAcc/1 -> Transfer Fcn/1
  Transfer Fcn/1 -> TF model/1

== system platoon/Vehicle 19 ==
  RefAcc : Inport
  i : Inport  Port=2
  Gain : Gain  Gain=-1*d_default
  Integrator : Integrator  InitialConditionSource=external
  TF model : cstblocks/LTI System  sys=G4  IC=[]
  Transfer Fcn : TransferFcn  Denominator=[td_input 1 0]
  position : Outport
  speed : Outport  Port=2
  wires:
  TF model/1 -> Integrator/1, speed/1
  Integrator/1 -> position/1
  i/1 -> Gain/1
  Gain/1 -> Integrator/2
  RefAcc/1 -> Transfer Fcn/1
  Transfer Fcn/1 -> TF model/1

== system platoon/Vehicle 2 ==
  RefAcc : Inport
  i : Inport  Port=2
  Gain : Gain  Gain=-1*d_default
  Integrator : Integrator  InitialConditionSource=external
  TF model : cstblocks/LTI System  sys=G4  IC=[]
  Transfer Fcn : TransferFcn  Denominator=[td_input 1 0]
  position : Outport
  speed : Outport  Port=2
  wires:
  TF model/1 -> Integrator/1, speed/1
  Integrator/1 -> position/1
  i/1 -> Gain/1
  Gain/1 -> Integrator/2
  RefAcc/1 -> Transfer Fcn/1
  Transfer Fcn/1 -> TF model/1

== system platoon/Vehicle 20 ==
  RefAcc : Inport
  i : Inport  Port=2
  Gain : Gain  Gain=-1*d_default
  Integrator : Integrator  InitialConditionSource=external
  TF model : cstblocks/LTI System  sys=G4  IC=[]
  Transfer Fcn : TransferFcn  Denominator=[td_input 1 0]
  position : Outport
  speed : Outport  Port=2
  wires:
  TF model/1 -> Integrator/1, speed/1
  Integrator/1 -> position/1
  i/1 -> Gain/1
  Gain/1 -> Integrator/2
  RefAcc/1 -> Transfer Fcn/1
  Transfer Fcn/1 -> TF model/1

== system platoon/Vehicle 3 ==
  RefAcc : Inport
  i : Inport  Port=2
  Gain : Gain  Gain=-1*d_default
  Integrator : Integrator  InitialConditionSource=external
  TF model : cstblocks/LTI System  sys=G4  IC=[]
  Transfer Fcn : TransferFcn  Denominator=[td_input 1 0]
  position : Outport
  speed : Outport  Port=2
  wires:
  TF model/1 -> Integrator/1, speed/1
  Integrator/1 -> position/1
  i/1 -> Gain/1
  Gain/1 -> Integrator/2
  RefAcc/1 -> Transfer Fcn/1
  Transfer Fcn/1 -> TF model/1

== system platoon/Vehicle 4 ==
  RefAcc : Inport
  i : Inport  Port=2
  Gain : Gain  Gain=-1*d_default
  Integrator : Integrator  InitialConditionSource=external
  TF model : cstblocks/LTI System  sys=G4  IC=[]
  Transfer Fcn : TransferFcn  Denominator=[td_input 1 0]
  position : Outport
  speed : Outport  Port=2
  wires:
  TF model/1 -> Integrator/1, speed/1
  Integrator/1 -> position/1
  i/1 -> Gain/1
  Gain/1 -> Integrator/2
  RefAcc/1 -> Transfer Fcn/1
  Transfer Fcn/1 -> TF model/1

== system platoon/Vehicle 5 ==
  RefAcc : Inport
  i : Inport  Port=2
  Gain : Gain  Gain=-1*d_default
  Integrator : Integrator  InitialConditionSource=external
  TF model : cstblocks/LTI System  sys=G4  IC=[]
  Transfer Fcn : TransferFcn  Denominator=[td_input 1 0]
  position : Outport
  speed : Outport  Port=2
  wires:
  TF model/1 -> Integrator/1, speed/1
  Integrator/1 -> position/1
  i/1 -> Gain/1
  Gain/1 -> Integrator/2
  RefAcc/1 -> Transfer Fcn/1
  Transfer Fcn/1 -> TF model/1

== system platoon/Vehicle 6 ==
  RefAcc : Inport
  i : Inport  Port=2
  Gain : Gain  Gain=-1*d_default
  Integrator : Integrator  InitialConditionSource=external
  TF model : cstblocks/LTI System  sys=G4  IC=[]
  Transfer Fcn : TransferFcn  Denominator=[td_input 1 0]
  position : Outport
  speed : Outport  Port=2
  wires:
  TF model/1 -> Integrator/1, speed/1
  Integrator/1 -> position/1
  i/1 -> Gain/1
  Gain/1 -> Integrator/2
  RefAcc/1 -> Transfer Fcn/1
  Transfer Fcn/1 -> TF model/1

== system platoon/Vehicle 7 ==
  RefAcc : Inport
  i : Inport  Port=2
  Gain : Gain  Gain=-1*d_default
  Integrator : Integrator  InitialConditionSource=external
  TF model : cstblocks/LTI System  sys=G4  IC=[]
  Transfer Fcn : TransferFcn  Denominator=[td_input 1 0]
  position : Outport
  speed : Outport  Port=2
  wires:
  TF model/1 -> Integrator/1, speed/1
  Integrator/1 -> position/1
  i/1 -> Gain/1
  Gain/1 -> Integrator/2
  RefAcc/1 -> Transfer Fcn/1
  Transfer Fcn/1 -> TF model/1

== system platoon/Vehicle 8 ==
  RefAcc : Inport
  i : Inport  Port=2
  Gain : Gain  Gain=-1*d_default
  Integrator : Integrator  InitialConditionSource=external
  TF model : cstblocks/LTI System  sys=G4  IC=[]
  Transfer Fcn : TransferFcn  Denominator=[td_input 1 0]
  position : Outport
  speed : Outport  Port=2
  wires:
  TF model/1 -> Integrator/1, speed/1
  Integrator/1 -> position/1
  i/1 -> Gain/1
  Gain/1 -> Integrator/2
  RefAcc/1 -> Transfer Fcn/1
  Transfer Fcn/1 -> TF model/1

== system platoon/Vehicle 9 ==
  RefAcc : Inport
  i : Inport  Port=2
  Gain : Gain  Gain=-1*d_default
  Integrator : Integrator  InitialConditionSource=external
  TF model : cstblocks/LTI System  sys=G4  IC=[]
  Transfer Fcn : TransferFcn  Denominator=[td_input 1 0]
  position : Outport
  speed : Outport  Port=2
  wires:
  TF model/1 -> Integrator/1, speed/1
  Integrator/1 -> position/1
  i/1 -> Gain/1
  Gain/1 -> Integrator/2
  RefAcc/1 -> Transfer Fcn/1
  Transfer Fcn/1 -> TF model/1

== system platoon/Subsystem1/Signal Builder New ==
  Demux : Demux  Tag=STV Demux  Outputs=1
      settings: DisplayOption=none
  FromWs : FromWorkspace  Tag=STV FromWs  VariableName=tuvar  SampleTime=0.001
      SigBuilderData=|
      | common.afterFinalStr = 'Extrapolate'
      | common.sampleTime = '0.001'
      | dataSet.timeRange = [0 120]
      | dataSet.name = 'Group 1'
      | sbobj.Groups.Name = 'Group 1'
      | sbobj.Groups.Signals.Name = 'Signal 1'
      | sbobj.Groups.Signals.XData = [0 2.5 5 7.5 10 12 13 15 30 34 40 45 60 64 74 80 84.2 90 94 100 102 120]
      | sbobj.Groups.Signals.YData = [0 4.5 4.5 0 0 -3 -3 0 0 -0.5 -0.5 1 1 0.5 0.5 -1 -1 -1.5 -1.5 -1 0 0]
      | sbobj.Groups.TimeRange = [0 120]
  Signal 1 : Outport  Tag=STV Outport  VectorParamsAs1DForOutWhenUnconnected=off
  wires:
  Demux/1 -> Signal 1/1
  FromWs/1 -> Demux/1
